simulink model "VZXA_DFPK_SA_MdlIdent"  (R2014b)
settings: Solver=ode45  StartTime=0.0  StopTime=147  MaxStep=.005  RelTol=1e-3
undefined symbols (not defined in the file or in its folder): mdlPara, PA_models_CMSI_piston_singleActing, PASL_Models
libraries: PASL_Pneumatics x6, PASL_Mechanics x2
settings Model: Creator=fbwk  LastModifiedBy=fbwk
settings DataIOCC: SaveOutput=off  SignalLogging=off  DSMLogging=off  SaveTime=off

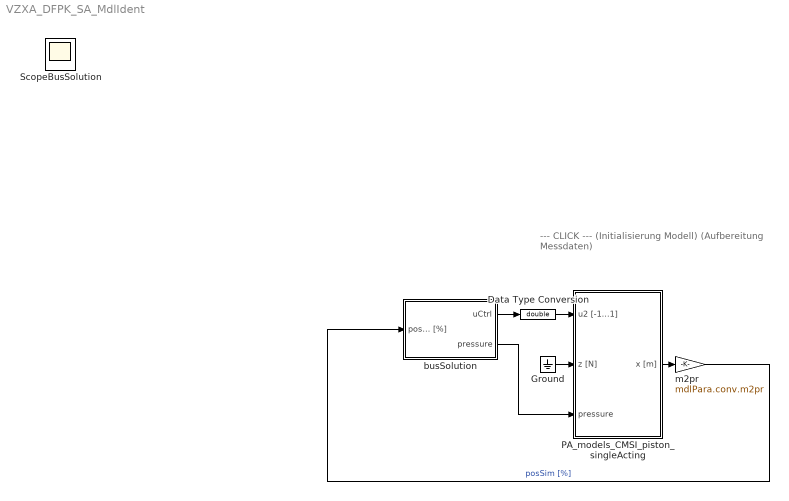
== system VZXA_DFPK_SA_MdlIdent ==
  note: --- CLICK ---
      | (Initialisierung Modell)
      | (Aufbereitung Messdaten)
  Data Type Conversion : DataTypeConversion  OutDataTypeStr=double
  Ground : Ground
  PA_models_CMSI_piston_singleActing : Subsystem  Tag=PA_models_CMSI_piston_singleActing  AncestorBlock=PASL_Models/PA_models_CMSI_piston_singleActing  mask(CMSI/Positioner Modell){mdlPara=mdlPara}
      mask prompts: mdlPara "Name of the parameters struct:"
      mask help:
      | Dieser Block beinhaltet das CMSI/Positioner Modell.
      |
      | Zur Initialisierung des Blocks kann entweder
      | a) ein vorhandener Parametersatz geladen werden
      | oder
      | b) ein default Datensatz generiert werden.
      | 	Dabei werden die Daten des CMSI/Positioners
      | 	abgefragt und alle aus der Konstruktion bekannten
      | 	Parameter entsprechend berechnet.
      | 	Für nicht bekannte Parameter wie z.B.
      | 	Reibung werden default Werte verwendet.
      |
      | 2015-08-28, fbwk
      mask Help: eval(['run(strcat(''',getenv('pasl_simulink'),''',''\documentation\tools\HelpForPaslElements.m''))']);
      mask DialogControl Control2 Prompt: PARAMETERSATZ LADEN
      mask DialogControl Control2 Callback:
      | try
      | 	%% Modellparameter %%%%%%%%%%%%%%%%%%%%%%%%%%%%%%%%%%%%%%%%%%%%%%%%%%%%%%%%
      | 	mdlParaDirectory = fullfile(getenv('pasl_simulink'),'PASL_Models\_mdlPara');
      | 	% choose and load dataset (change local directories here)
      | 	dlgTitle = 'Which dataset?';
      | 	dlgDefAns = [mdlParaDirectory,'\mdlPara_Positioner_optim_17.mat'];
      | 	% UI for selecting dataset
      | 	[datasetName, datasetPath] = uigetfile( ...
      | 		[mdlParaDirectory,'\mdlPara*.mat'], ...
      | 		dlgTitle,dlgDefAns,'MultiSelect', 'off');
      | 	% load dataset
      | 		disp(['  - load model parameters from ''', datasetName, ''' ...'])
      | 	load([datasetPath,datasetName])
      | catch
      | 	disp('WARNING: ')
      | 	disp('Could not load parameter set.')
      | end
      | 
      | % clear section
      | clear mdlParaDirectory dlgTitle dlgDefAns datasetName datasetPath
      mask DialogControl Control3 Prompt: default Werte generieren
      mask DialogControl Control3 Callback: run(fullfile(getenv('pasl_simulink'),'PASL_Models\_mdlPara','aux_initMdlParaPositioner'))
      mask Display:
      | image(imread('FestoProzVent.png'))
      | 
      | port_label('input',1,'u2 [-1...1]')
      | port_label('input',2,'z [N]')
      | port_label('output',1,'x [m]')
  busSolution : Subsystem  VariantControl=busVariant
  m2pr : Gain  Gain=mdlPara.conv.m2pr  OutDataTypeStr=single
  ScopeBusSolution : Scope  NumInputPorts=5
      settings: ShowLegends=on  TimeRange=147  YMin=-10~-100~-1.1~90000~-1.1  YMax=110~20~1.1~850000~1.1
  wires:
  Ground/1 -> PA_models_CMSI_piston_singleActing/2(z [N])
  Data Type Conversion/1 -> PA_models_CMSI_piston_singleActing/1(u2 [-1...1])
  m2pr/1 -> busSolution/1(posSim [%])  "posSim [%]"
  PA_models_CMSI_piston_singleActing/1(x [m]) -> m2pr/1
  busSolution/1(uCtrl) -> Data Type Conversion/1
  busSolution/2(pressure) -> PA_models_CMSI_piston_singleActing/3(pressure)

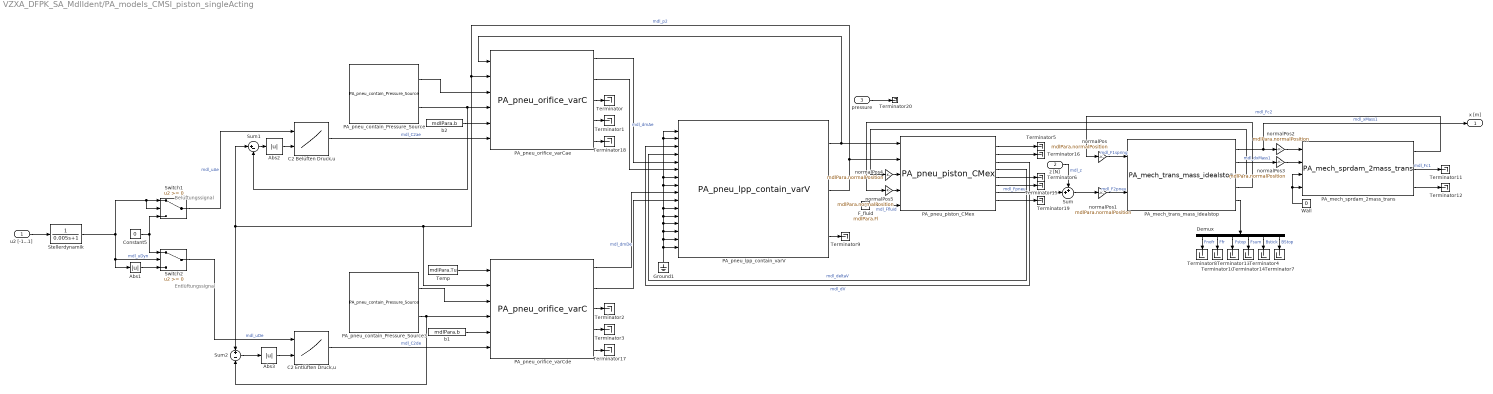
== system VZXA_DFPK_SA_MdlIdent/PA_models_CMSI_piston_singleActing ==
  note: Entlüftungssignal
  note: Belüftungssignal
  u2 [-1...1] : Inport
  z [N] : Inport  Port=2
  pressure : Inport  Port=3
  Abs1 : Abs
  Abs2 : Abs
  Abs3 : Abs
  C2 Belüften Druck,u : Lookup_n-D  BreakpointsForDimension1=mdlPara.C2.u  BreakpointsForDimension2=mdlPara.C2.deltap  Table=mdlPara.C2.ae  ExtrapMethod=Clip  UseLastTableValue=on  InternalRulePriority=Speed  RndMeth=Simplest  InputSameDT=on
  C2 Entlüften Druck,u : Lookup_n-D  BreakpointsForDimension1=mdlPara.C2.u  BreakpointsForDimension2=mdlPara.C2.deltap  Table=mdlPara.C2.de  ExtrapMethod=Clip  UseLastTableValue=on  InternalRulePriority=Speed  RndMeth=Simplest  InputSameDT=on
  Constant5 : Constant  Value=0
  Demux : Demux  Outputs=6
  F_fluid : Constant  Value=mdlPara.Fl
  Ground1 : Ground
  PA_mech_sprdam_2mass_trans : PASL_Mechanics/Spring and Damping Elements/PA_mech_sprdam_2mass_trans  Tag=PA_mech_sprdam_2mass_trans  ctrans=mdlPara.c  dtrans=mdlPara.d  x0=mdlPara.xfZero  lot=0
  PA_mech_trans_mass_idealstop : PASL_Mechanics/Moving Masses/PA_mech_trans_mass_idealstop  Tag=RB_mech_trans_mass_idealstop  xinit=mdlPara.x0  xdotinit=mdlPara.v0  m=mdlPara.mass  dtrans1=mdlPara.viscFriCoeff1  dtrans2=mdlPara.viscFriCoeff2  dtrans3=mdlPara.viscFriCoeff3  xdotstri=mdlPara.stribeckVel  Fstick=mdlPara.Fstick  Fslip=mdlPara.Fcoulomb  xmin=mdlPara.xMin  xmax=mdlPara.xMax
  PA_pneu_contain_Pressure_Source : PASL_Pneumatics/Volumes/PA_pneu_contain_Pressure_Source  Tag=FE_pneu_contain_Env  T0=mdlPara.Tu  p0=mdlPara.pv  sourcetype=automatic mode
  PA_pneu_contain_Pressure_Source3 : PASL_Pneumatics/Volumes/PA_pneu_contain_Pressure_Source  Tag=FE_pneu_contain_Env  T0=mdlPara.Tu  p0=mdlPara.pu  sourcetype=automatic mode
  PA_pneu_lpp_contain_varV : PASL_Pneumatics/Volumes/PA_pneu_lpp_contain_varV  p0=mdlPara.p02  T0=mdlPara.Tu  V0=mdlPara.V02  K=mdlPara.heatExCoeff  A=mdlPara.heatExArea  Tw=mdlPara.Tu  R=mdlPara.R  kappa=mdlPara.kappa  temp_effects=without temperature effects
  PA_pneu_orifice_varCae : PASL_Pneumatics/Orifices/PA_pneu_orifice_varC  Tag=FE_pneu_orifice_VarA  R=mdlPara.R  kappa=mdlPara.kappa  p0=mdlPara.pu  T0=mdlPara.Tu  Smooth_fact=mdlPara.smoothFac  temp_effects=with temperature effects
  PA_pneu_orifice_varCde : PASL_Pneumatics/Orifices/PA_pneu_orifice_varC  Tag=FE_pneu_orifice_VarA  R=mdlPara.R  kappa=mdlPara.kappa  p0=mdlPara.pu  T0=mdlPara.Tu  Smooth_fact=mdlPara.smoothFac  temp_effects=with temperature effects
  PA_pneu_piston_CMex : PASL_Pneumatics/Pistons/PA_pneu_piston_CMex  d_out=mdlPara.d2Out  d_in=mdlPara.d2In  p0=mdlPara.pu  x_0=mdlPara.x0
  Stellerdynamik : TransferFcn  Denominator=[0.005 1]
  Sum : Sum  Inputs=++|
  Sum1 : Sum  Inputs=|+-
  Sum2 : Sum  Inputs=+|-
  Switch1 : Switch
  Switch2 : Switch
  Temp : Constant  Value=mdlPara.Tu
  Terminator{,1..20} (21 alike) : Terminator
  Wall : Constant  Value=0
  b1 : Constant  Value=mdlPara.b
  b2 : Constant  Value=mdlPara.b
  normalPos{,1..5} (6 alike) : Gain  Gain=mdlPara.normalPosition
  x [m] : Outport
  wires:
  z [N]/1 -> Sum/1  "mdl_z"
  PA_pneu_piston_CMex/4 -> PA_pneu_lpp_contain_varV/4  "mdl_deltaV"
  PA_pneu_piston_CMex/3 -> PA_pneu_lpp_contain_varV/3  "mdl_dV"
  PA_pneu_piston_CMex/7 -> Sum/2  "mdl_Fpneu"
  PA_pneu_lpp_contain_varV/3 -> Terminator9/1
  Demux/6 -> Terminator7/1  "BStop"
  Demux/5 -> Terminator4/1  "Bstick"
  Demux/4 -> Terminator14/1  "Fsum"
  Demux/3 -> Terminator13/1  "Fstop"
  Demux/2 -> Terminator10/1  "Ffr"
  Demux/1 -> Terminator8/1  "Fnofr"
  Stellerdynamik/1 -> Switch2/2, Abs1/1, Switch1/1, Switch1/2  "mdl_uDyn"
  Temp/1 -> PA_pneu_orifice_varCde/1
  Switch1/1 -> C2 Belüften Druck,u/1  "mdl_uAe"
  u2 [-1...1]/1 -> Stellerdynamik/1
  Switch2/1 -> C2 Entlüften Druck,u/1  "mdl_uDe"
  Constant5/1 -> Switch1/3, Switch2/1
  Abs1/1 -> Switch2/3
  F_fluid/1 -> PA_pneu_piston_CMex/5  "mdl_Ffluid"
  PA_pneu_piston_CMex/2 -> Terminator16/1
  PA_pneu_piston_CMex/1 -> Terminator5/1
  PA_pneu_piston_CMex/8 -> Terminator19/1
  Wall/1 -> PA_mech_sprdam_2mass_trans/3, PA_mech_sprdam_2mass_trans/4
  PA_mech_trans_mass_idealstop/5 -> Demux/1
  PA_mech_trans_mass_idealstop/2 -> normalPos3/1  "mdl_dxMass1"
  PA_mech_trans_mass_idealstop/1 -> normalPos2/1, x [m]/1  "mdl_xMass1"
  PA_mech_sprdam_2mass_trans/1 -> normalPos/1  "mdl_Fc2"
  PA_mech_sprdam_2mass_trans/2 -> Terminator11/1  "mdl_Fc1"
  PA_mech_sprdam_2mass_trans/3 -> Terminator12/1
  PA_pneu_orifice_varCae/5 -> Terminator18/1
  PA_pneu_orifice_varCde/5 -> Terminator17/1
  b2/1 -> PA_pneu_orifice_varCae/5
  b1/1 -> PA_pneu_orifice_varCde/5
  PA_pneu_piston_CMex/6 -> Terminator15/1
  PA_pneu_piston_CMex/5 -> Terminator6/1
  Ground1/1 -> PA_pneu_lpp_contain_varV/2, PA_pneu_lpp_contain_varV/1, PA_pneu_lpp_contain_varV/7, PA_pneu_lpp_contain_varV/8, PA_pneu_lpp_contain_varV/11, PA_pneu_lpp_contain_varV/12, PA_pneu_lpp_contain_varV/13, PA_pneu_lpp_contain_varV/14, PA_pneu_lpp_contain_varV/15, PA_pneu_lpp_contain_varV/16
  PA_pneu_orifice_varCde/4 -> Terminator3/1
  PA_pneu_orifice_varCde/3 -> Terminator2/1
  PA_pneu_orifice_varCae/4 -> Terminator1/1
  PA_pneu_orifice_varCae/3 -> Terminator/1
  PA_pneu_orifice_varCde/2 -> PA_pneu_lpp_contain_varV/10  "mdl_dmDe"
  PA_pneu_orifice_varCde/1 -> PA_pneu_lpp_contain_varV/9
  PA_pneu_contain_Pressure_Source3/2 -> Sum2/2, PA_pneu_orifice_varCde/4
  PA_pneu_contain_Pressure_Source3/1 -> PA_pneu_orifice_varCde/3
  PA_pneu_contain_Pressure_Source/2 -> Sum1/2, PA_pneu_orifice_varCae/4
  PA_pneu_contain_Pressure_Source/1 -> PA_pneu_orifice_varCae/3
  PA_pneu_lpp_contain_varV/2 -> PA_pneu_orifice_varCae/2, Sum1/1, Sum2/1, PA_pneu_orifice_varCde/2, PA_pneu_piston_CMex/2  "mdl_p2"
  PA_pneu_lpp_contain_varV/1 -> PA_pneu_piston_CMex/1, PA_pneu_orifice_varCae/1
  PA_pneu_orifice_varCae/2 -> PA_pneu_lpp_contain_varV/6  "mdl_dmAe"
  PA_pneu_orifice_varCae/1 -> PA_pneu_lpp_contain_varV/5
  C2 Belüften Druck,u/1 -> PA_pneu_orifice_varCae/6  "mdl_C2ae"
  C2 Entlüften Druck,u/1 -> PA_pneu_orifice_varCde/6  "mdl_C2de"
  Sum2/1 -> Abs3/1
  Abs3/1 -> C2 Entlüften Druck,u/2
  Sum1/1 -> Abs2/1
  Abs2/1 -> C2 Belüften Druck,u/2
  Sum/1 -> normalPos1/1
  PA_mech_trans_mass_idealstop/3 -> normalPos4/1
  PA_mech_trans_mass_idealstop/4 -> normalPos5/1
  normalPos1/1 -> PA_mech_trans_mass_idealstop/2  "mdl_F2pneu"
  normalPos4/1 -> PA_pneu_piston_CMex/3
  normalPos5/1 -> PA_pneu_piston_CMex/4
  normalPos/1 -> PA_mech_trans_mass_idealstop/1  "mdl_F1spring"
  normalPos2/1 -> PA_mech_sprdam_2mass_trans/1
  normalPos3/1 -> PA_mech_sprdam_2mass_trans/2
  pressure/1 -> Terminator20/1

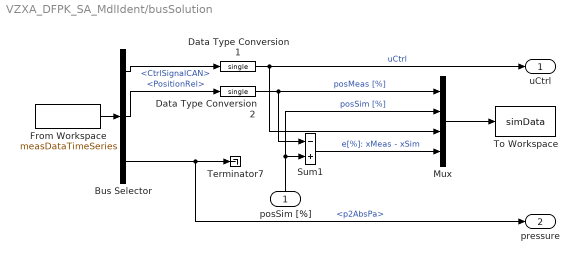
== system VZXA_DFPK_SA_MdlIdent/busSolution ==
  posSim [%] : Inport
  Bus Selector : BusSelector  OutputSignals=CtrlSignalCAN,PositionRel,p2AbsPa
  Data Type Conversion1 : DataTypeConversion  OutDataTypeStr=single
  Data Type Conversion2 : DataTypeConversion  OutDataTypeStr=single
  From Workspace : FromWorkspace  VariableName=measDataTimeSeries  OutDataTypeStr=Bus: busMeasData  SampleTime=0
  Mux : Mux
  Sum1 : Sum  Inputs=-+
  Terminator7 : Terminator
  To Workspace : ToWorkspace  VariableName=simData  SaveFormat=Structure With Time  SampleTime=-1
  uCtrl : Outport
  pressure : Outport  Port=2
  wires:
  Bus Selector/3 -> pressure/1, Terminator7/1  "<p2AbsPa>"
  Bus Selector/1 -> Data Type Conversion1/1  "<CtrlSignalCAN>"
  From Workspace/1 -> Bus Selector/1
  Bus Selector/2 -> Data Type Conversion2/1  "<PositionRel>"
  posSim [%]/1 -> Mux/2, Sum1/2  "posSim [%]"
  Sum1/1 -> Mux/4  "e[%]: xMeas - xSim"
  Mux/1 -> To Workspace/1
  Data Type Conversion1/1 -> Mux/3, uCtrl/1  "uCtrl"
  Data Type Conversion2/1 -> Sum1/1, Mux/1  "posMeas [%]"
